simulink model "lineerFollowerModel"  (R2021a)
settings: Solver=ode23  StartTime=0.0  StopTime=1000  RelTol=1e-3
model workspace (MAT data in the model file):
  SL_ROS_VariableLengthArrays_MaxSizes : object (value not decoded)
values from neighbouring files (symbols this model uses):
  A_1 = linsys1.A    [AssignMatrices.m]
  B_1 = linsys1.B    [AssignMatrices.m]
  C_1 = linsys1.C    [AssignMatrices.m]
  D_1 = linsys1.D    [AssignMatrices.m]
  u0_Thrust = fileName.Inputs(4).u    [AssignMatrices.m]
  u1max = deg2rad(25)    [AssignMatrices.m]
  u1min = deg2rad(-25)    [AssignMatrices.m]
  u2max = deg2rad(10)    [AssignMatrices.m]
  u2min = deg2rad(-25)    [AssignMatrices.m]
  u3max = deg2rad(30)    [AssignMatrices.m]
  u3min = deg2rad(-30)    [AssignMatrices.m]
undefined symbols (not defined in the file or in its folder): ModelName, ModelName_SL_Info, Pose, sigbuilder_block
libraries: pid_lib x16, robotlib x7, robotcorelib x1, sharedtransform x1, simulink_extras x1
(part 2 of 2)

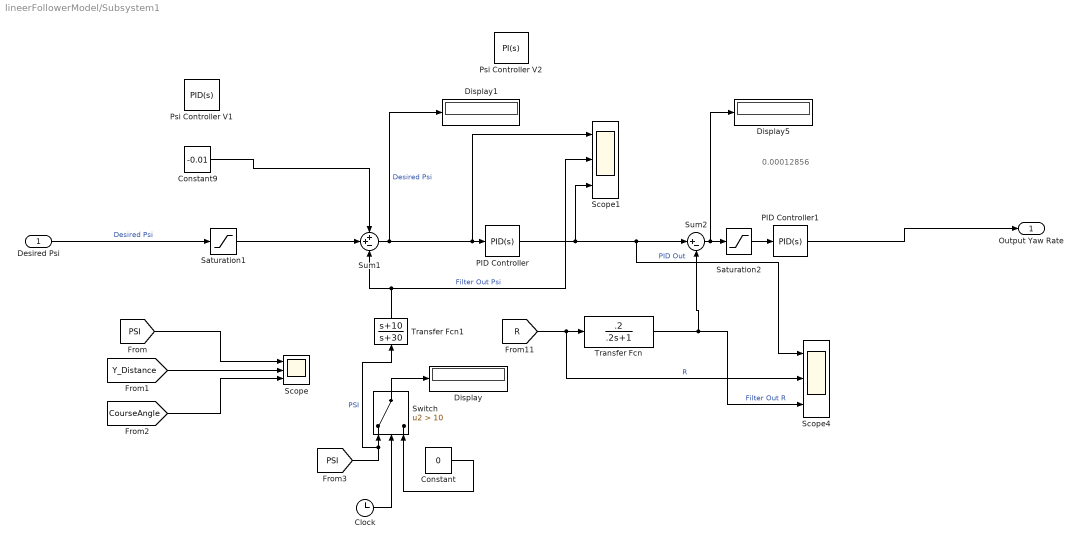
== system lineerFollowerModel/Subsystem1 ==
  note: 0.00012856
  "Desired Psi " : Inport
  Clock : Clock
  Constant : Constant  Value=0
  Constant9 : Constant  Value=-0.01
  Display : Display
  Display1 : Display
  Display5 : Display
  PID Controller : pid_lib/PID Controller  Controller=PID  Form=Parallel  TimeDomain=Continuous-time  UseExternalTs=off  SampleTime=-1  IntegratorMethod=Forward Euler  FilterMethod=Forward Euler  ControllerParametersSource=internal  P=1  I=7e-7  D=50  UseFilter=on  N=1  TunerSelectOption=Transfer Function Based (PID Tuner App)  InitialConditionSource=internal  InitialConditionForIntegrator=0  InitialConditionForFilter=0  DifferentiatorICPrevScaledInput=0  ExternalReset=none  TrackingMode=off  Kt=1  LimitOutput=off  SatLimitsSource=internal  UpperSaturationLimit=inf  LowerSaturationLimit=-inf  LinearizeAsGain=on  AntiWindupMode=none  Kb=1  POutMin=[]  POutMax=[]  IOutMin=[]  IOutMax=[]  DOutMin=[]  DOutMax=[]  NOutMin=[]  NOutMax=[]  SumOutMin=[]  SumOutMax=[]  SaturationOutMin=[]  SaturationOutMax=[]  PParamMin=[]  PParamMax=[]  IParamMin=[]  IParamMax=[]  DParamMin=[]  DParamMax=[]  NParamMin=[]  NParamMax=[]  KbParamMin=[]  KbParamMax=[]  KtParamMin=[]  KtParamMax=[]  KbOutMin=[]  KbOutMax=[]  KtOutMin=[]  KtOutMax=[]  IntegratorOutMin=[]  IntegratorOutMax=[]  FilterOutMin=[]  FilterOutMax=[]  SumI1OutMin=[]  SumI1OutMax=[]  SumI2OutMin=[]  SumI2OutMax=[]  SumI3OutMin=[]  SumI3OutMax=[]  SumI4OutMin=[]  SumI4OutMax=[]  SumDOutMin=[]  SumDOutMax=[]  DifferentiatorOutMin=[]  DifferentiatorOutMax=[]  FilterDiffOutCoefMin=[]  FilterDiffOutCoefMax=[]  ReciprocalOutMin=[]  ReciprocalOutMax=[]  SumDenOutMin=[]  SumDenOutMax=[]  SumNumOutMin=[]  SumNumOutMax=[]  DivideOutMin=[]  DivideOutMax=[]  UdiffTsProdOutMin=[]  UdiffTsProdOutMax=[]  NTsProdOutMin=[]  NTsProdOutMax=[]  UintegralTsProdOutMin=[]  UintegralTsProdOutMax=[]  UngainTsProdOutMin=[]  UngainTsProdOutMax=[]  IntegratorContinuousStateAttributes=''  IntegratorStateMustResolveToSignalObject=off  IntegratorRTWStateStorageClass=Auto  FilterContinuousStateAttributes=''  FilterStateMustResolveToSignalObject=off  FilterRTWStateStorageClass=Auto  ParallelPVariant=InternalParameters  IdealPVariant=Disabled  IVariant=InternalParameters  DVariant=InternalParameters  IntegratorVariant=Continuous  SatVariant=Disabled  AWVariant=Passthrough  PCopyVariant=Disabled  TRVariant=Disabled  FdbkBlocksVariant=Forward  IdealPFdbkVariant=Disabled  SatFdbkVariant=Disabled  DerivativeFilterVariant=ContFilter  NVariant=InternalParameters  NCopyVariant=Disabled  FilterICVariant=InternalICsFilter  IntegratorICVariant=InternalICs  ExternalResetVariant=Disabled  TRSumVariant=Passthrough  SumFdbkVariant=Disabled  SumVariant=Sum_PID  TsampFilterVariant=InternalTs  TsampNgainVariant=Passthrough  TsampIntegralVariant=Passthrough  ExternalSaturationOutDataTypeStr=Inherit: Same as second input
  PID Controller1 : pid_lib/PID Controller  Controller=PID  Form=Parallel  TimeDomain=Continuous-time  UseExternalTs=off  SampleTime=-1  IntegratorMethod=Forward Euler  FilterMethod=Forward Euler  ControllerParametersSource=internal  P=-1.84519165653966  I=-7.75213296090846e-04  D=933.217701780908  UseFilter=on  N=0.000396560228767529  TunerSelectOption=Transfer Function Based (PID Tuner App)  InitialConditionSource=internal  InitialConditionForIntegrator=0  InitialConditionForFilter=0  DifferentiatorICPrevScaledInput=0  ExternalReset=none  TrackingMode=off  Kt=1  LimitOutput=off  SatLimitsSource=internal  UpperSaturationLimit=inf  LowerSaturationLimit=-inf  LinearizeAsGain=on  AntiWindupMode=none  Kb=1  POutMin=[]  POutMax=[]  IOutMin=[]  IOutMax=[]  DOutMin=[]  DOutMax=[]  NOutMin=[]  NOutMax=[]  SumOutMin=[]  SumOutMax=[]  SaturationOutMin=[]  SaturationOutMax=[]  PParamMin=[]  PParamMax=[]  IParamMin=[]  IParamMax=[]  DParamMin=[]  DParamMax=[]  NParamMin=[]  NParamMax=[]  KbParamMin=[]  KbParamMax=[]  KtParamMin=[]  KtParamMax=[]  KbOutMin=[]  KbOutMax=[]  KtOutMin=[]  KtOutMax=[]  IntegratorOutMin=[]  IntegratorOutMax=[]  FilterOutMin=[]  FilterOutMax=[]  SumI1OutMin=[]  SumI1OutMax=[]  SumI2OutMin=[]  SumI2OutMax=[]  SumI3OutMin=[]  SumI3OutMax=[]  SumI4OutMin=[]  SumI4OutMax=[]  SumDOutMin=[]  SumDOutMax=[]  DifferentiatorOutMin=[]  DifferentiatorOutMax=[]  FilterDiffOutCoefMin=[]  FilterDiffOutCoefMax=[]  ReciprocalOutMin=[]  ReciprocalOutMax=[]  SumDenOutMin=[]  SumDenOutMax=[]  SumNumOutMin=[]  SumNumOutMax=[]  DivideOutMin=[]  DivideOutMax=[]  UdiffTsProdOutMin=[]  UdiffTsProdOutMax=[]  NTsProdOutMin=[]  NTsProdOutMax=[]  UintegralTsProdOutMin=[]  UintegralTsProdOutMax=[]  UngainTsProdOutMin=[]  UngainTsProdOutMax=[]  IntegratorContinuousStateAttributes=''  IntegratorStateMustResolveToSignalObject=off  IntegratorRTWStateStorageClass=Auto  FilterContinuousStateAttributes=''  FilterStateMustResolveToSignalObject=off  FilterRTWStateStorageClass=Auto  ParallelPVariant=InternalParameters  IdealPVariant=Disabled  IVariant=InternalParameters  DVariant=InternalParameters  IntegratorVariant=Continuous  SatVariant=Disabled  AWVariant=Passthrough  PCopyVariant=Disabled  TRVariant=Disabled  FdbkBlocksVariant=Forward  IdealPFdbkVariant=Disabled  SatFdbkVariant=Disabled  DerivativeFilterVariant=ContFilter  NVariant=InternalParameters  NCopyVariant=Disabled  FilterICVariant=InternalICsFilter  IntegratorICVariant=InternalICs  ExternalResetVariant=Disabled  TRSumVariant=Passthrough  SumFdbkVariant=Disabled  SumVariant=Sum_PID  TsampFilterVariant=InternalTs  TsampNgainVariant=Passthrough  TsampIntegralVariant=Passthrough  ExternalSaturationOutDataTypeStr=Inherit: Same as second input
  Psi Controller V1 : pid_lib/PID Controller  Controller=PID  Form=Parallel  TimeDomain=Continuous-time  UseExternalTs=off  SampleTime=-1  IntegratorMethod=Forward Euler  FilterMethod=Forward Euler  ControllerParametersSource=internal  P=50.0840046771307  I=7.11153544700578e-02  D=200  UseFilter=on  N=0.000923562844274157  TunerSelectOption=Transfer Function Based (PID Tuner App)  InitialConditionSource=internal  InitialConditionForIntegrator=0  InitialConditionForFilter=0  DifferentiatorICPrevScaledInput=0  ExternalReset=none  TrackingMode=off  Kt=1  LimitOutput=off  SatLimitsSource=internal  UpperSaturationLimit=inf  LowerSaturationLimit=-inf  LinearizeAsGain=on  AntiWindupMode=none  Kb=1  POutMin=[]  POutMax=[]  IOutMin=[]  IOutMax=[]  DOutMin=[]  DOutMax=[]  NOutMin=[]  NOutMax=[]  SumOutMin=[]  SumOutMax=[]  SaturationOutMin=[]  SaturationOutMax=[]  PParamMin=[]  PParamMax=[]  IParamMin=[]  IParamMax=[]  DParamMin=[]  DParamMax=[]  NParamMin=[]  NParamMax=[]  KbParamMin=[]  KbParamMax=[]  KtParamMin=[]  KtParamMax=[]  KbOutMin=[]  KbOutMax=[]  KtOutMin=[]  KtOutMax=[]  IntegratorOutMin=[]  IntegratorOutMax=[]  FilterOutMin=[]  FilterOutMax=[]  SumI1OutMin=[]  SumI1OutMax=[]  SumI2OutMin=[]  SumI2OutMax=[]  SumI3OutMin=[]  SumI3OutMax=[]  SumI4OutMin=[]  SumI4OutMax=[]  SumDOutMin=[]  SumDOutMax=[]  DifferentiatorOutMin=[]  DifferentiatorOutMax=[]  FilterDiffOutCoefMin=[]  FilterDiffOutCoefMax=[]  ReciprocalOutMin=[]  ReciprocalOutMax=[]  SumDenOutMin=[]  SumDenOutMax=[]  SumNumOutMin=[]  SumNumOutMax=[]  DivideOutMin=[]  DivideOutMax=[]  UdiffTsProdOutMin=[]  UdiffTsProdOutMax=[]  NTsProdOutMin=[]  NTsProdOutMax=[]  UintegralTsProdOutMin=[]  UintegralTsProdOutMax=[]  UngainTsProdOutMin=[]  UngainTsProdOutMax=[]  IntegratorContinuousStateAttributes=''  IntegratorStateMustResolveToSignalObject=off  IntegratorRTWStateStorageClass=Auto  FilterContinuousStateAttributes=''  FilterStateMustResolveToSignalObject=off  FilterRTWStateStorageClass=Auto  ParallelPVariant=InternalParameters  IdealPVariant=Disabled  IVariant=InternalParameters  DVariant=InternalParameters  IntegratorVariant=Continuous  SatVariant=Disabled  AWVariant=Passthrough  PCopyVariant=Disabled  TRVariant=Disabled  FdbkBlocksVariant=Forward  IdealPFdbkVariant=Disabled  SatFdbkVariant=Disabled  DerivativeFilterVariant=ContFilter  NVariant=InternalParameters  NCopyVariant=Disabled  FilterICVariant=InternalICsFilter  IntegratorICVariant=InternalICs  ExternalResetVariant=Disabled  TRSumVariant=Passthrough  SumFdbkVariant=Disabled  SumVariant=Sum_PID  TsampFilterVariant=InternalTs  TsampNgainVariant=Passthrough  TsampIntegralVariant=Passthrough  ExternalSaturationOutDataTypeStr=Inherit: Same as second input
  Psi Controller V2 : pid_lib/PID Controller  Controller=PI  Form=Parallel  TimeDomain=Continuous-time  UseExternalTs=off  SampleTime=-1  IntegratorMethod=Forward Euler  FilterMethod=Forward Euler  ControllerParametersSource=internal  P=1  I=7e-7  D=50  UseFilter=on  N=0.000923562844274157  TunerSelectOption=Transfer Function Based (PID Tuner App)  InitialConditionSource=internal  InitialConditionForIntegrator=0  InitialConditionForFilter=0  DifferentiatorICPrevScaledInput=0  ExternalReset=none  TrackingMode=off  Kt=1  LimitOutput=off  SatLimitsSource=internal  UpperSaturationLimit=inf  LowerSaturationLimit=-inf  LinearizeAsGain=on  AntiWindupMode=none  Kb=1  POutMin=[]  POutMax=[]  IOutMin=[]  IOutMax=[]  DOutMin=[]  DOutMax=[]  NOutMin=[]  NOutMax=[]  SumOutMin=[]  SumOutMax=[]  SaturationOutMin=[]  SaturationOutMax=[]  PParamMin=[]  PParamMax=[]  IParamMin=[]  IParamMax=[]  DParamMin=[]  DParamMax=[]  NParamMin=[]  NParamMax=[]  KbParamMin=[]  KbParamMax=[]  KtParamMin=[]  KtParamMax=[]  KbOutMin=[]  KbOutMax=[]  KtOutMin=[]  KtOutMax=[]  IntegratorOutMin=[]  IntegratorOutMax=[]  FilterOutMin=[]  FilterOutMax=[]  SumI1OutMin=[]  SumI1OutMax=[]  SumI2OutMin=[]  SumI2OutMax=[]  SumI3OutMin=[]  SumI3OutMax=[]  SumI4OutMin=[]  SumI4OutMax=[]  SumDOutMin=[]  SumDOutMax=[]  DifferentiatorOutMin=[]  DifferentiatorOutMax=[]  FilterDiffOutCoefMin=[]  FilterDiffOutCoefMax=[]  ReciprocalOutMin=[]  ReciprocalOutMax=[]  SumDenOutMin=[]  SumDenOutMax=[]  SumNumOutMin=[]  SumNumOutMax=[]  DivideOutMin=[]  DivideOutMax=[]  UdiffTsProdOutMin=[]  UdiffTsProdOutMax=[]  NTsProdOutMin=[]  NTsProdOutMax=[]  UintegralTsProdOutMin=[]  UintegralTsProdOutMax=[]  UngainTsProdOutMin=[]  UngainTsProdOutMax=[]  IntegratorContinuousStateAttributes=''  IntegratorStateMustResolveToSignalObject=off  IntegratorRTWStateStorageClass=Auto  FilterContinuousStateAttributes=''  FilterStateMustResolveToSignalObject=off  FilterRTWStateStorageClass=Auto  ParallelPVariant=InternalParameters  IdealPVariant=Disabled  IVariant=InternalParameters  DVariant=Disabled  IntegratorVariant=Continuous  SatVariant=Disabled  AWVariant=Passthrough  PCopyVariant=Disabled  TRVariant=Disabled  FdbkBlocksVariant=Forward  IdealPFdbkVariant=Disabled  SatFdbkVariant=Disabled  DerivativeFilterVariant=Disabled  NVariant=Disabled  NCopyVariant=Disabled_SignalSpec  FilterICVariant=Disabled  IntegratorICVariant=InternalICs  ExternalResetVariant=Disabled  TRSumVariant=Passthrough  SumFdbkVariant=Disabled  SumVariant=Sum_PI  TsampFilterVariant=InternalTs  TsampNgainVariant=Passthrough  TsampIntegralVariant=Passthrough  ExternalSaturationOutDataTypeStr=Inherit: Same as second input
  Saturation1 : Saturate  UpperLimit=0.65  LowerLimit=-0.1
  Saturation2 : Saturate  UpperLimit=u3max  LowerLimit=u3min
  Scope : Scope  NumInputPorts=3
  Scope1 : Scope  NumInputPorts=3
  Scope4 : Scope  NumInputPorts=3
  Sum1 : Sum  Inputs=++-
  Sum2 : Sum  Inputs=|+-
  Switch : Switch  Criteria=u2 > Threshold  Threshold=10
  Transfer Fcn : TransferFcn  Numerator=[.2]  Denominator=[.2 1]
  Transfer Fcn1 : TransferFcn  Numerator=[1 10 ]  Denominator=[1 30]
  Output Yaw Rate : Outport
  wires:
  PID Controller1/1 -> Output Yaw Rate/1
  Saturation2/1 -> PID Controller1/1
  Transfer Fcn/1 -> Scope4/3, Sum2/2  "Filter Out R"
  Sum2/1 -> Display5/1, Saturation2/1
  [R] -> Scope4/2, Transfer Fcn/1  "R"
  [PSI] -> Scope/1
  [Y_Distance] -> Scope/2
  [CourseAngle] -> Scope/3
  Sum1/1 -> Scope1/1, PID Controller/1, Display1/1  "Desired Psi"
  PID Controller/1 -> Scope4/1, Sum2/1, Scope1/3  "PID Out"
  "Desired Psi "/1 -> Saturation1/1  "Desired Psi"
  Transfer Fcn1/1 -> Sum1/3, Scope1/2  "Filter Out Psi"
  Clock/1 -> Switch/2
  Switch/1 -> Display/1
  [PSI] -> Transfer Fcn1/1, Switch/1  "PSI"
  Constant/1 -> Switch/3
  Saturation1/1 -> Sum1/2
  Constant9/1 -> Sum1/1

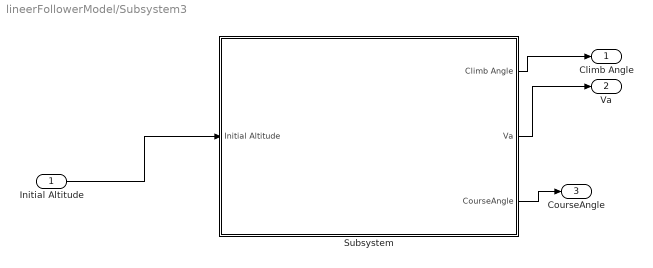
== system lineerFollowerModel/Subsystem3 ==
  Initial Altitude : Inport
  Subsystem : Subsystem
  Climb Angle : Outport
  Va : Outport  Port=2
  CourseAngle : Outport  Port=3
  wires:
  Subsystem/1(Climb Angle) -> Climb Angle/1
  Subsystem/2(Va) -> Va/1
  Subsystem/3(CourseAngle) -> CourseAngle/1
  Initial Altitude/1 -> Subsystem/1(Initial Altitude)

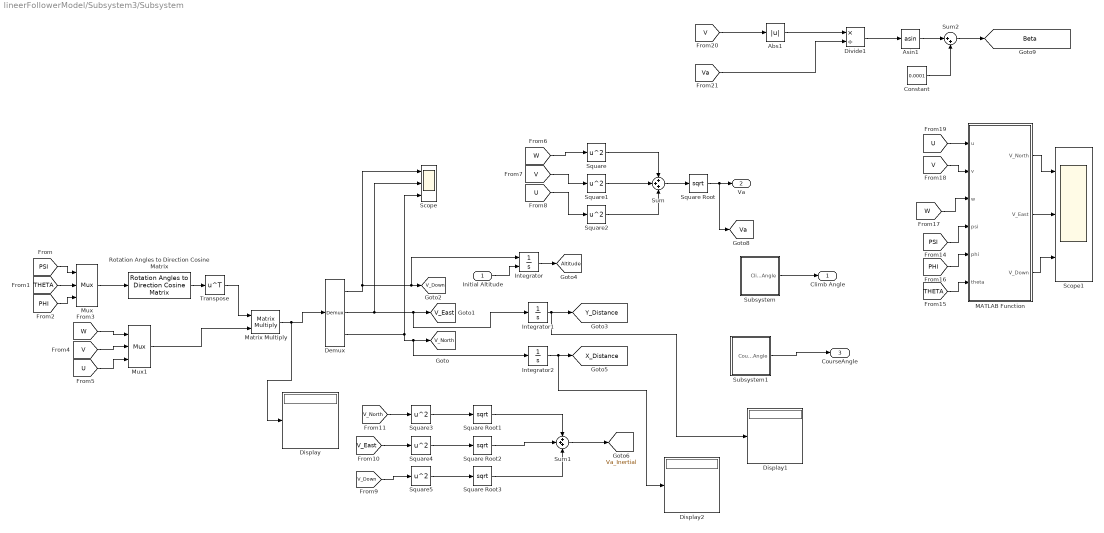
== system lineerFollowerModel/Subsystem3/Subsystem ==
  Initial Altitude : Inport
  Abs1 : Abs
  Asin1 : Trigonometry  Operator=asin
  Constant : Constant  Value=0.0001
  Demux : Demux  Outputs=3
  Display : Display
  Display1 : Display
  Display2 : Display
  Divide1 : Product  Inputs=*/
  Integrator : Integrator  InitialConditionSource=external  LowerSaturationLimit=0
  Integrator1 : Integrator  UpperSaturationLimit=+10  LowerSaturationLimit=-10
  Integrator2 : Integrator  LimitOutput=on
  MATLAB Function : MATLAB Function  TreatAsAtomicUnit=on
  Matrix Multiply : Product  Multiplication=Matrix(*)
  Mux : Mux  Inputs=3
  Mux1 : Mux  Inputs=3
  Rotation Angles to Direction Cosine Matrix : sharedtransform/Rotation Angles to Direction Cosine Matrix  rotationOrder=ZYX  aMode=aMode
      settings: SourceProductBaseCode=AE,PW,MT,UV,VE,VP
  Scope : Scope  NumInputPorts=3
  Scope1 : Scope  NumInputPorts=3
  Square{,1..5} (6 alike) : Math  Operator=square  SaturateOnIntegerOverflow=on
  Square Root{,1..3} (4 alike) : Sqrt  SaturateOnIntegerOverflow=on
  Subsystem : Subsystem
  Subsystem1 : Subsystem
  Sum : Sum  Inputs=+++
  Sum1 : Sum  Inputs=+++
  Sum2 : Sum  Inputs=|++
  Transpose : Math  Operator=transpose  SignedPower=on  SaturateOnIntegerOverflow=on
  Climb Angle : Outport
  Va : Outport  Port=2
  CourseAngle : Outport  Port=3
  tag scope: Altitude=global, Beta=global, V_Down=global, V_East=global, V_North=global, Va=global, Va_Inertial=global, X_Distance=global, Y_Distance=global
  wires:
  Square1/1 -> Sum/2
  Square Root/1 -> [Va], Va/1
  Sum/1 -> Square Root/1
  Square2/1 -> Sum/3
  Square/1 -> Sum/1
  Subsystem/1(Climb Angle) -> Climb Angle/1
  Rotation Angles to Direction Cosine Matrix/1 -> Transpose/1
  Mux/1 -> Rotation Angles to Direction Cosine Matrix/1
  Transpose/1 -> Matrix Multiply/1
  Mux1/1 -> Matrix Multiply/2
  Matrix Multiply/1 -> Display/1, Demux/1
  Demux/1 -> Integrator/1, [V_Down], Scope/1
  Demux/2 -> Integrator1/1, [V_East], Scope/2
  Demux/3 -> Integrator2/1, [V_North], Scope/3
  [PSI] -> Mux/1
  [PHI] -> Mux/3
  [THETA] -> Mux/2
  [W] -> Mux1/1
  [V] -> Mux1/2
  [U] -> Mux1/3
  [W] -> Square/1
  [V] -> Square1/1
  [U] -> Square2/1
  Subsystem1/1(CourseAngle) -> CourseAngle/1
  Initial Altitude/1 -> Integrator/2
  Integrator1/1 -> Display1/1, [Y_Distance]
  Integrator2/1 -> Display2/1, [X_Distance]
  [V_Down] -> Square5/1
  [V_East] -> Square4/1
  [V_North] -> Square3/1
  Square5/1 -> Square Root3/1
  Square4/1 -> Square Root2/1
  Square3/1 -> Square Root1/1
  Square Root1/1 -> Sum1/1
  Square Root2/1 -> Sum1/2
  Square Root3/1 -> Sum1/3
  Sum1/1 -> [Va_Inertial]
  [PHI] -> MATLAB Function/5(phi)
  [PSI] -> MATLAB Function/4(psi)
  [THETA] -> MATLAB Function/6(theta)
  [U] -> MATLAB Function/1(u)
  [V] -> MATLAB Function/2(v)
  [W] -> MATLAB Function/3(w)
  MATLAB Function/1(V_North) -> Scope1/1
  MATLAB Function/2(V_East) -> Scope1/2
  MATLAB Function/3(V_Down) -> Scope1/3
  Integrator/1 -> [Altitude]
  Abs1/1 -> Divide1/1
  Divide1/1 -> Asin1/1
  [V] -> Abs1/1
  [Va] -> Divide1/2
  Sum2/1 -> [Beta]
  Asin1/1 -> Sum2/1
  Constant/1 -> Sum2/2

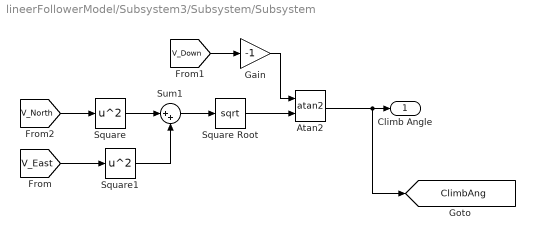
== system lineerFollowerModel/Subsystem3/Subsystem/Subsystem ==
  Atan2 : Trigonometry  Operator=atan2
  Gain : Gain  Gain=-1
  Square : Math  Operator=square  SaturateOnIntegerOverflow=on
  Square Root : Sqrt  SaturateOnIntegerOverflow=on
  Square1 : Math  Operator=square  SaturateOnIntegerOverflow=on
  Sum1 : Sum  Inputs=|++
  Climb Angle : Outport
  tag scope: ClimbAng=global
  wires:
  Atan2/1 -> [ClimbAng], Climb Angle/1
  [V_North] -> Square/1
  [V_East] -> Square1/1
  Square/1 -> Sum1/1
  Square1/1 -> Sum1/2
  Sum1/1 -> Square Root/1
  Square Root/1 -> Atan2/2
  [V_Down] -> Gain/1
  Gain/1 -> Atan2/1

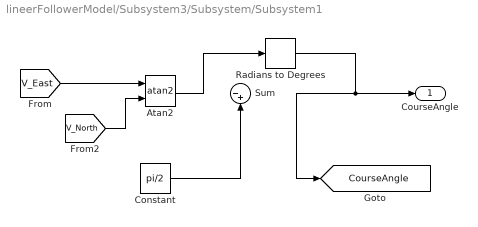
== system lineerFollowerModel/Subsystem3/Subsystem/Subsystem1 ==
  Atan2 : Trigonometry  Operator=atan2
  Constant : Constant  Value=pi/2
  Radians to Degrees : simulink_extras/Transformations/Radians to Degrees
  Sum : Sum  Inputs=|-+
  CourseAngle : Outport
  tag scope: CourseAngle=global
  wires:
  Constant/1 -> Sum/2
  [V_East] -> Atan2/1
  [V_North] -> Atan2/2
  Atan2/1 -> Radians to Degrees/1
  Radians to Degrees/1 -> [CourseAngle], CourseAngle/1

== matlab function lineerFollowerModel/Subsystem3/Subsystem/MATLAB Function ==
  data: u input; V_North output; v input; w input; psi input; phi input; theta input; V_East output; V_Down output
function [V_North, V_East, V_Down] = fcn(u,v,w,psi,phi,theta)

% V_North = u*(cos(theta)*cos(psi)) + v*(sin(phi)*sin(theta)*cos(psi)- cos(phi)*sin(psi)) + w*(cos(phi)*sin(theta)*cos(psi)+sin(phi)*sin(psi));
% V_East = u*(cos(theta)*sin(psi)) + v*(sin(phi)*sin(theta)*sin(psi) + cos(phi)*cos(psi)) + w*(cos(phi)*sin(theta)*cos(psi)-sin(phi)*cos(psi));
% V_Down = u*(-sin(theta)) + v*(sin(phi)*cos(theta)) + w*(cos(phi)*cos(theta));

x7 = phi;
x8 = theta;
x9 = psi;

V_b = [u;v;w];

C12 = [cos(x9) -sin(x9) 0;
        sin(x9) cos(x9) 0;
        0 0 1];
C23 = [cos(x8) 0 sin(x8);
        0 1 0;
        -sin(x8) 0 cos(x8)];
C3i = [1 0 0;
    0 cos(x7) -sin(x7);
    0 sin(x7) cos(x7)];


Cvb = C12*C23*C3i; 

V_Earth = Cvb * V_b;

V_North = V_Earth(1);
V_East = V_Earth(2);
V_Down = V_Earth(3);

== matlab function lineerFollowerModel/MATLAB Function ==
  data: y output; data input
function y = fcn(data)

[centersDark,radiiDark] = imfindcircles(data,[10 300],'ObjectPolarity','dark', 'Sensitivity',0.92);

if ~isempty(centersDark)
    xPos = -5.983*10^-7*radiiDark(1)^5 + 0.0001086*radiiDark(1)^4 - 0.00788*radiiDark(1)^3 + 0.292*radiiDark(1)^2 - 5.812*radiiDark(1) + 59;
    yPos = (320-centersDark(1))/(2*radiiDark(1));
    zPos = (240-centersDark(2))/(1.5*radiiDark(1));
else
    xPos = 0;
    yPos = 0;
    zPos = 0;
end
if ~isempty(centersDark) && centersDark(1) < 320
    yPos = -yPos;
end
if ~isempty(centersDark) && centersDark(2) > 240
    zPos = -zPos;
end
y = [ xPos yPos zPos ];
